simulink model "untitled"  (R2018b)
settings: Solver=VariableStepAuto  StartTime=0.0  StopTime=10.0  RelTol=1e-3
settings Model: Creator=AYDIN  LastModifiedBy=AYDIN

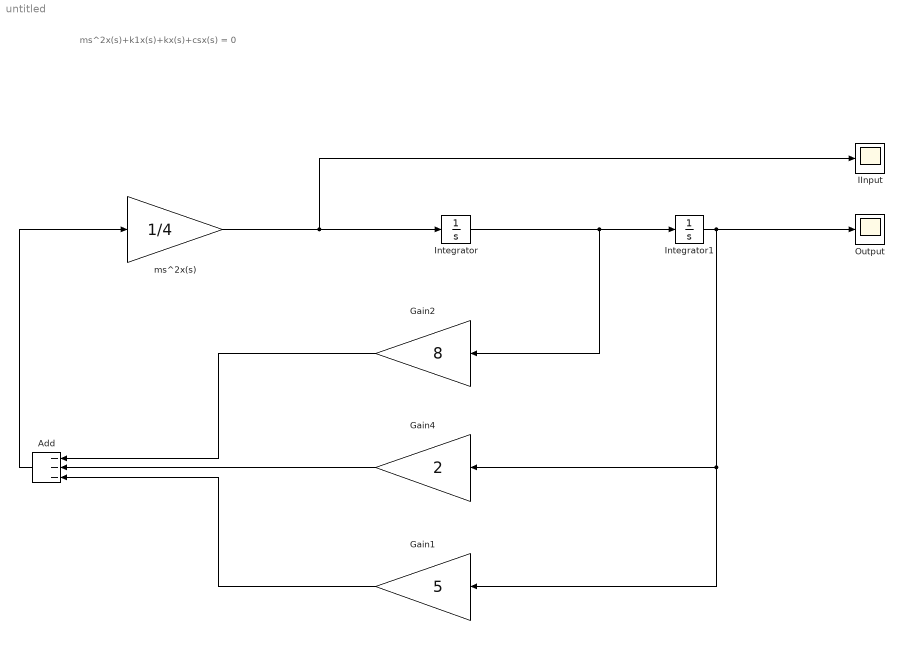
== system untitled ==
  note: ms^2x(s)+k1x(s)+kx(s)+csx(s) = 0
  Add : Sum  Inputs=---
  Gain1 : Gain  Gain=5
  Gain2 : Gain  Gain=8
  Gain4 : Gain  Gain=2
  "IInput " : Scope
  Integrator : Integrator
  Integrator1 : Integrator  InitialCondition=0.6
  "Output " : Scope
  ms^2x(s) : Gain  Gain=1/4
  wires:
  ms^2x(s)/1 -> "IInput "/1, Integrator/1
  Integrator/1 -> Gain2/1, Integrator1/1
  Integrator1/1 -> "Output "/1, Gain4/1, Gain1/1
  Gain4/1 -> Add/2
  Gain2/1 -> Add/1
  Gain1/1 -> Add/3
  Add/1 -> ms^2x(s)/1
